simulink model "tanques_Hinf_fenom_w1w2"  (R2015a)
settings: Solver=ode45  StartTime=0.0  StopTime=t_run/Ts_fen  RelTol=1e-3
values from neighbouring files (symbols this model uses):
  Ak = Phi_amp + H*C_amp + Gamma_amp*Ck    [Hinf_LSDP_ident.m]    (also in Hinf_LSDP_pheno.m; Quad_tank_Hinf_LSDP_control_pheno.m; Quad_tank_Hinf_LSDP_control_phenoW1W2.m; Quad_tank_Hinf_LSDP_control_phenoW1W2_ident.m)
  Bk = -H + Gamma_amp*Dk    [Hinf_LSDP_ident.m]    (also in Hinf_LSDP_pheno.m; Quad_tank_Hinf_LSDP_control_pheno.m; Quad_tank_Hinf_LSDP_control_phenoW1W2.m; Quad_tank_Hinf_LSDP_control_phenoW1W2_ident.m)
  Ck = F2 - Dk*(C_amp + Z2\F1)    [Hinf_LSDP_ident.m]    (also in Hinf_LSDP_pheno.m; Quad_tank_Hinf_LSDP_control_pheno.m; Quad_tank_Hinf_LSDP_control_phenoW1W2.m; Quad_tank_Hinf_LSDP_control_phenoW1W2_ident.m)
  Dk = (eye(2) + Gamma_amp.'*Xinf*Gamma_amp)\Gamma_amp.'*Xinf*H    [Hinf_LSDP_ident.m]    (also in Hinf_LSDP_pheno.m; Quad_tank_Hinf_LSDP_control_pheno.m; Quad_tank_Hinf_LSDP_control_phenoW1W2.m; Quad_tank_Hinf_LSDP_control_phenoW1W2_ident.m)
  hinicial = [9 7 0 0]    [Hinf_LSDP_ident.m]    (also in Hinf_LSDP_pheno.m; Model.m = [hi1 hi2 0 0]; Modelo.m = [hi1 hi2 0 0]; Quad_tank_Hinf_LSDP_control_pheno.m = [7 7 0 0])
  SYS_d = c2d(SYS_c,Ts)    [Hinf_LSDP_ident.m]    (also in Hinf_LSDP_pheno.m; Quad_tank_Hinf_LSDP_control_pheno.m = c2d(SYS_c,Ts_fen); Quad_tank_Hinf_LSDP_control_phenoW1W2.m = c2d(SYS_c,Ts_fen); Quad_tank_Hinf_LSDP_control_phenoW1W2_ident.m = c2d(SYS_c,Ts_fen))
  sys_W1_d = ss(c2d(W1,Ts),'minimal')    [Hinf_LSDP_ident.m]    (also in Hinf_LSDP_pheno.m; Quad_tank_Hinf_LSDP_control_phenoW1W2.m = ss(c2d(W1,Ts_fen),'minimal'); Quad_tank_Hinf_LSDP_control_phenoW1W2_ident.m)
  Ts = 0.1    [Hinf_LSDP_ident.m]    (also in Hinf_LSDP_pheno.m; Quad_tank_Hinf_LSDP_control_pheno.m = 1; Quad_tank_Hinf_LSDP_control_phenoW1W2.m = 1; Quad_tank_Hinf_LSDP_control_phenoW1W2_ident.m = 1)
  Ts_fen = 0.1    [Quad_tank_Hinf_LSDP_control_pheno.m]    (also in Quad_tank_Hinf_LSDP_control_phenoW1W2.m; Quad_tank_Hinf_LSDP_control_phenoW1W2_ident.m)
settings Model: Creator=pcosta  LastModifiedBy=plinio

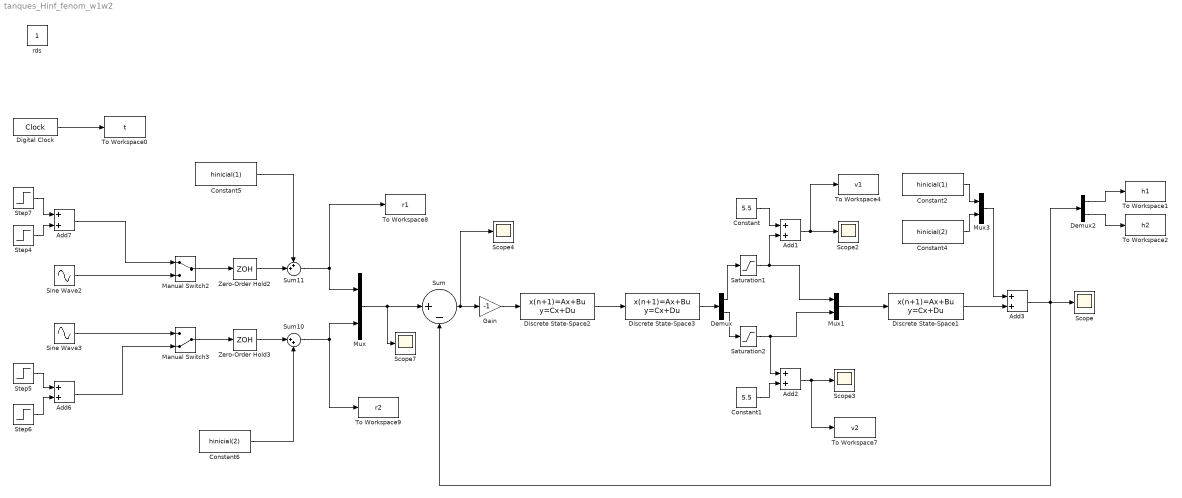
== system tanques_Hinf_fenom_w1w2 ==
  Add{1..3,6..7} (5 alike) : Sum
  Constant : Constant  Value=5.5
  Constant1 : Constant  Value=5.5
  Constant2 : Constant  Value=hinicial(1)
  Constant4 : Constant  Value=hinicial(2)
  Constant5 : Constant  Value=hinicial(1)
  Constant6 : Constant  Value=hinicial(2)
  Demux : Demux  Outputs=2
  Demux2 : Demux  Outputs=2
  Digital Clock : DigitalClock  SampleTime=Ts
  Discrete State-Space1 : DiscreteStateSpace  A=SYS_d.a  B=SYS_d.b  C=SYS_d.c  D=SYS_d.d  SampleTime=Ts_fen
  Discrete State-Space2 : DiscreteStateSpace  A=Ak  B=Bk  C=Ck  D=Dk
  Discrete State-Space3 : DiscreteStateSpace  A=sys_W1_d.a  B=sys_W1_d.b  C=sys_W1_d.c  D=sys_W1_d.d  SampleTime=Ts
  Gain : Gain  Gain=-1
  Manual Switch2 : ManualSwitch
  Manual Switch3 : ManualSwitch  CurrentSetting=0
  Mux : Mux  Inputs=2
  Mux1 : Mux  Inputs=2
  Mux3 : Mux  Inputs=2
  Saturation1 : Saturate  UpperLimit=4.5  LowerLimit=-5.5
  Saturation2 : Saturate  UpperLimit=4.5  LowerLimit=-5.5
  Scope{,2..4,7} (5 alike) : Scope
      Scope settings: MaxDataPoints=5000000
      Scope2 settings: SaveName=ScopeData2  MaxDataPoints=500000
      Scope3 settings: SaveName=ScopeData3  MaxDataPoints=500000
      Scope4 settings: SaveName=ScopeData4
      Scope7 settings: SaveName=ScopeData7
  Sine Wave2 : Sin  Frequency=0.1  SampleTime=0
  Sine Wave3 : Sin  Frequency=0.1  Phase=pi/2  SampleTime=0
  Step4 : Step  Time=400/Ts_fen  After=-3  SampleTime=Ts_fen  ZeroCross=off
  Step5 : Step  Time=200/Ts_fen  After=3  SampleTime=Ts_fen  ZeroCross=off
  Step6 : Step  Time=600/Ts_fen  After=-3  SampleTime=Ts_fen  ZeroCross=off
  Step7 : Step  Time=10/Ts_fen  After=3  SampleTime=Ts_fen  ZeroCross=off
  Sum : Sum  Inputs=|+-
  Sum10 : Sum  Inputs=|++
  Sum11 : Sum  Inputs=++|
  To Workspace0 : ToWorkspace  VariableName=t  SampleTime=-1
  To Workspace1 : ToWorkspace  VariableName=h1  SampleTime=-1
  To Workspace2 : ToWorkspace  VariableName=h2  SampleTime=-1
  To Workspace4 : ToWorkspace  VariableName=v1  SampleTime=-1
  To Workspace7 : ToWorkspace  VariableName=v2  SampleTime=-1
  To Workspace8 : ToWorkspace  VariableName=r1  SampleTime=-1
  To Workspace9 : ToWorkspace  VariableName=r2  SampleTime=-1
  Zero-Order Hold2 : ZeroOrderHold  SampleTime=Ts
  Zero-Order Hold3 : ZeroOrderHold  SampleTime=Ts
  rds : Constant  IOType=siggen
  wires:
  Mux/1 -> Scope7/1, Sum/1
  Constant/1 -> Add1/1
  Add1/1 -> Scope2/1, To Workspace4/1
  Add2/1 -> Scope3/1, To Workspace7/1
  Constant1/1 -> Add2/2
  Demux2/1 -> To Workspace1/1
  Demux2/2 -> To Workspace2/1
  Digital Clock/1 -> To Workspace0/1
  Sum/1 -> Scope4/1, Gain/1
  Constant6/1 -> Sum10/2
  Step4/1 -> Add7/2
  Step7/1 -> Add7/1
  Constant5/1 -> Sum11/1
  Step5/1 -> Add6/1
  Step6/1 -> Add6/2
  Add7/1 -> Manual Switch2/1
  Sine Wave2/1 -> Manual Switch2/2
  Sine Wave3/1 -> Manual Switch3/1
  Add6/1 -> Manual Switch3/2
  Zero-Order Hold3/1 -> Sum10/1
  Constant2/1 -> Mux3/1
  Constant4/1 -> Mux3/2
  Mux3/1 -> Add3/1
  Manual Switch2/1 -> Zero-Order Hold2/1
  Manual Switch3/1 -> Zero-Order Hold3/1
  Sum10/1 -> To Workspace9/1, Mux/2
  Discrete State-Space1/1 -> Add3/2
  Sum11/1 -> Mux/1, To Workspace8/1
  Zero-Order Hold2/1 -> Sum11/2
  Add3/1 -> Sum/2, Demux2/1, Scope/1
  Gain/1 -> Discrete State-Space2/1
  Discrete State-Space2/1 -> Discrete State-Space3/1
  Discrete State-Space3/1 -> Demux/1
  Saturation1/1 -> Mux1/1, Add1/2
  Demux/1 -> Saturation1/1
  Demux/2 -> Saturation2/1
  Saturation2/1 -> Add2/1, Mux1/2
  Mux1/1 -> Discrete State-Space1/1
